simulink model "INDI_POS_SMC_Att"  (R2024b)
settings: Solver=FixedStepDiscrete  StartTime=0.0  StopTime=70  FixedStep=1/250  RelTol=1e-3
values from neighbouring files (symbols this model uses):
  acc_gain = diag([0.5   0.5   0.3  ])    [Parameter.m]
  g = 9.8067    [Parameter.m]
  Jx = 0.005    [Parameter.m]
  Jy = 0.005    [Parameter.m]
  Jz = 0.009    [Parameter.m]
  K2 = 0    [Parameter.m]
  k5 = 0.0388    [Parameter.m]
  k6 = 0.0219    [Parameter.m]
  k7 = 0.3147    [Parameter.m]
  k8 = 0.1244    [Parameter.m]
  l = 0.165    [Parameter.m]
  m = 0.8    [Parameter.m]
  pos_gain = diag([4.14  4.14  3.105])    [Parameter.m]
  Qmax = 0.05    [Parameter.m]
  Tmax = 4    [Parameter.m]
  vel_gain = diag([2.34  2.34  1.77 ])    [Parameter.m]
undefined symbols (not defined in the file or in its folder): DiscIntNeverNeededParam
libraries: simulink x4
settings Model: Creator=user  LastModifiedBy=user
settings DebuggingCC: AlgebraicLoopMsg=none

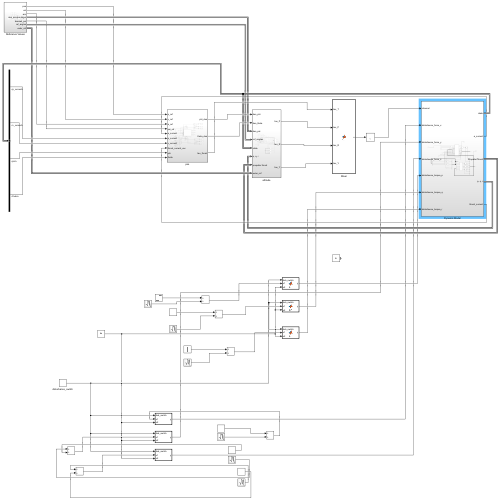
[thumbnail: Simulink's stored preview of the top-level diagram]
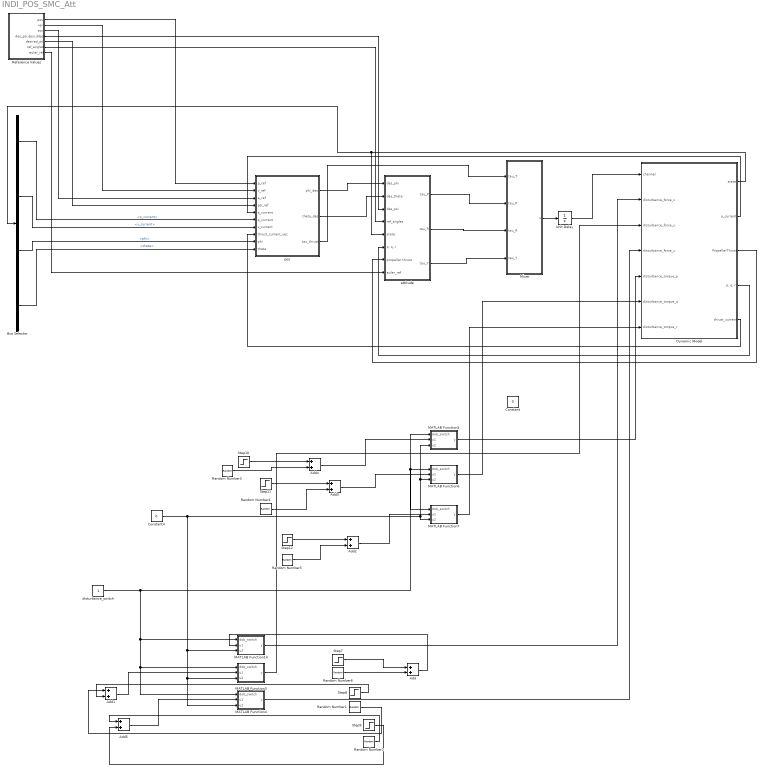
== system INDI_POS_SMC_Att ==
  Add{,1..5} (6 alike) : Sum
  Bus Selector : BusSelector  OutputSignals=p_current,v_current,phi,theta
  Constant : Constant  Value=0
  Constant4 : Constant  Value=0  SampleTime=-1
  Dynamic Model : Subsystem
  MATLAB Function14 : MATLAB Function  TreatAsAtomicUnit=on
  MATLAB Function3 : MATLAB Function  TreatAsAtomicUnit=on
  MATLAB Function4 : MATLAB Function  TreatAsAtomicUnit=on
  MATLAB Function5 : MATLAB Function  TreatAsAtomicUnit=on
  MATLAB Function6 : MATLAB Function  TreatAsAtomicUnit=on
  MATLAB Function7 : MATLAB Function  TreatAsAtomicUnit=on
  Mixer : MATLAB Function  TreatAsAtomicUnit=on
  Random Number{1..6} (6 alike) : RandomNumber  Variance=0.1
  Reference Values : Subsystem
  Step10 : Step  Time=0  After=15
  Step11 : Step  Time=0  After=-15
  Step12 : Step  Time=0  After=2
  Step7 : Step  Time=0
  Step8 : Step  Time=0  After=-0.5
  Step9 : Step  Time=0  After=5
  Unit Delay : UnitDelay  SampleTime=-1  HasFrameUpgradeWarning=on
  attitude : Subsystem
  disturbance_switch : Constant  SampleTime=-1
  pos : Subsystem
  wires:
  Reference Values/1(pos) -> pos/1(p_ref)
  Reference Values/2(vel) -> pos/2(v_ref)
  Reference Values/3(acc) -> pos/3(a_ref)
  Reference Values/5(desired_psi) -> pos/4(psi_ref)
  Bus Selector/1 -> pos/6(p_current)  "<p_current>"
  Bus Selector/2 -> pos/7(v_current)  "<v_current>"
  Reference Values/6(ref_angles) -> attitude/4(ref_angles)
  pos/1(phi_des) -> attitude/1(des_phi)
  pos/2(theta_des) -> attitude/2(des_theta)
  Reference Values/4(des_psi,dpsi,ddpsi) -> attitude/3(des_psi)
  Mixer/1(u) -> Unit Delay/1
  Random Number5/1 -> Add2/2
  Add3/1 -> MATLAB Function6/2(u1)
  Constant4/1 -> MATLAB Function5/3(u2), MATLAB Function6/3(u2), MATLAB Function7/3(u2), MATLAB Function4/3(u2), MATLAB Function3/3(u2), MATLAB Function14/3(u2)
  Step10/1 -> Add4/1
  Add2/1 -> MATLAB Function7/2(u1)
  Random Number4/1 -> Add3/2
  Step11/1 -> Add3/1
  Random Number3/1 -> Add4/2
  disturbance_switch/1 -> MATLAB Function5/1(dob_switch), MATLAB Function7/1(dob_switch), MATLAB Function6/1(dob_switch), MATLAB Function14/1(dob_switch), MATLAB Function4/1(dob_switch), MATLAB Function3/1(dob_switch)
  Add4/1 -> MATLAB Function5/2(u1)
  Step12/1 -> Add2/1
  Step7/1 -> Add/1
  Step8/1 -> Add1/2
  Random Number6/1 -> Add/2
  Step9/1 -> Add5/2
  Add/1 -> MATLAB Function14/2(u1)
  Add1/1 -> MATLAB Function3/2(u1)
  Add5/1 -> MATLAB Function4/2(u1)
  Random Number2/1 -> Add5/1
  Random Number1/1 -> Add1/1
  pos/3(tau_thrust) -> Mixer/1(tau_T)
  attitude/1(tau_P) -> Mixer/2(tau_P)
  attitude/2(tau_R) -> Mixer/3(tau_R)
  attitude/3(tau_Y) -> Mixer/4(tau_Y)
  Dynamic Model/1(state) -> Bus Selector/1, attitude/5(state)
  Dynamic Model/2(a_current) -> pos/5(a_current)
  Dynamic Model/3(PropellerThrust) -> attitude/7(propeller thrust)
  Dynamic Model/4("p, q, r") -> attitude/6("p, q, r")
  Dynamic Model/5(thrust_current) -> pos/8(thrust_current_vec)
  Bus Selector/3 -> pos/9(phi)  "<phi>"
  Bus Selector/4 -> pos/10(theta)  "<theta>"
  MATLAB Function14/1(y) -> Dynamic Model/2(disturbance_force_x)
  MATLAB Function3/1(y) -> Dynamic Model/3(disturbance_force_y)
  MATLAB Function4/1(y) -> Dynamic Model/4(disturbance_force_z)
  MATLAB Function5/1(y) -> Dynamic Model/5(disturbance_torque_p)
  MATLAB Function6/1(y) -> Dynamic Model/6(disturbance_torque_q)
  MATLAB Function7/1(y) -> Dynamic Model/7(disturbance_torque_r)
  Reference Values/7(euler_ref) -> attitude/8(euler_ref)
  Unit Delay/1 -> Dynamic Model/1(channel)

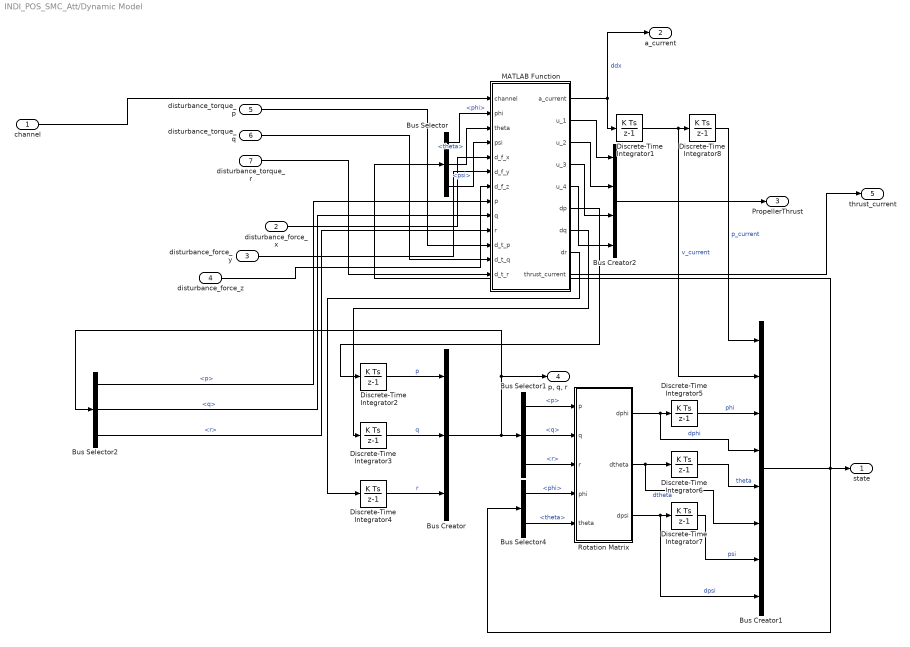
== system INDI_POS_SMC_Att/Dynamic Model ==
  channel : Inport
  disturbance_force_x : Inport  Port=2
  disturbance_force_y : Inport  Port=3
  disturbance_force_z : Inport  Port=4
  disturbance_torque_p : Inport  Port=5
  disturbance_torque_q : Inport  Port=6
  disturbance_torque_r : Inport  Port=7
  Bus Creator : BusCreator  Inputs=3
  Bus Creator1 : BusCreator  Inputs=8
  Bus Creator2 : BusCreator  Inputs=4
  Bus Selector : BusSelector  OutputSignals=phi,theta,psi
  Bus Selector1 : BusSelector  OutputSignals=p,q,r
  Bus Selector2 : BusSelector  OutputSignals=p,q,r
  Bus Selector4 : BusSelector  OutputSignals=phi,theta
  Discrete-Time Integrator{1..8} (8 alike) : DiscreteIntegrator  SampleTime=-1  ICPrevOutput=DiscIntNeverNeededParam  ICPrevScaledInput=DiscIntNeverNeededParam
  MATLAB Function : MATLAB Function  TreatAsAtomicUnit=on
  Rotation Matrix : MATLAB Function  TreatAsAtomicUnit=on
  state : Outport
  a_current : Outport  Port=2
  PropellerThrust : Outport  Port=3
  "p, q, r" : Outport  Port=4
  thrust_current : Outport  Port=5
  wires:
  disturbance_force_y/1 -> MATLAB Function/6(d_f_y)
  disturbance_force_z/1 -> MATLAB Function/7(d_f_z)
  disturbance_force_x/1 -> MATLAB Function/5(d_f_x)
  channel/1 -> MATLAB Function/1(channel)
  Discrete-Time Integrator2/1 -> Bus Creator/1  "p"
  Discrete-Time Integrator3/1 -> Bus Creator/2  "q"
  Discrete-Time Integrator4/1 -> Bus Creator/3  "r"
  Bus Selector2/1 -> MATLAB Function/8(p)  "<p>"
  Bus Selector2/2 -> MATLAB Function/9(q)  "<q>"
  Bus Selector2/3 -> MATLAB Function/10(r)  "<r>"
  Bus Selector1/1 -> Rotation Matrix/1(p)  "<p>"
  Bus Selector1/2 -> Rotation Matrix/2(q)  "<q>"
  Bus Selector1/3 -> Rotation Matrix/3(r)  "<r>"
  Bus Selector4/1 -> Rotation Matrix/4(phi)  "<phi>"
  Bus Selector4/2 -> Rotation Matrix/5(theta)  "<theta>"
  Rotation Matrix/1(dphi) -> Bus Creator1/4, Discrete-Time Integrator5/1  "dphi"
  Rotation Matrix/2(dtheta) -> Bus Creator1/6, Discrete-Time Integrator6/1  "dtheta"
  Rotation Matrix/3(dpsi) -> Bus Creator1/8, Discrete-Time Integrator7/1  "dpsi"
  Discrete-Time Integrator5/1 -> Bus Creator1/3  "phi"
  Discrete-Time Integrator6/1 -> Bus Creator1/5  "theta"
  Discrete-Time Integrator7/1 -> Bus Creator1/7  "psi"
  Discrete-Time Integrator1/1 -> Bus Creator1/2, Discrete-Time Integrator8/1  "v_current"
  Discrete-Time Integrator8/1 -> Bus Creator1/1  "p_current"
  Bus Selector/1 -> MATLAB Function/2(phi)  "<phi>"
  Bus Selector/2 -> MATLAB Function/3(theta)  "<theta>"
  Bus Selector/3 -> MATLAB Function/4(psi)  "<psi>"
  MATLAB Function/2(u_1) -> Bus Creator2/1
  MATLAB Function/3(u_2) -> Bus Creator2/2
  MATLAB Function/4(u_3) -> Bus Creator2/3
  MATLAB Function/5(u_4) -> Bus Creator2/4
  Bus Creator2/1 -> PropellerThrust/1
  disturbance_torque_q/1 -> MATLAB Function/12(d_t_q)
  disturbance_torque_r/1 -> MATLAB Function/13(d_t_r)
  disturbance_torque_p/1 -> MATLAB Function/11(d_t_p)
  MATLAB Function/6(dp) -> Discrete-Time Integrator2/1
  MATLAB Function/7(dq) -> Discrete-Time Integrator3/1
  MATLAB Function/8(dr) -> Discrete-Time Integrator4/1
  Bus Creator/1 -> Bus Selector1/1, Bus Selector2/1, "p, q, r"/1
  Bus Creator1/1 -> Bus Selector/1, Bus Selector4/1, state/1
  MATLAB Function/1(a_current) -> a_current/1, Discrete-Time Integrator1/1  "ddx"
  MATLAB Function/9(thrust_current) -> thrust_current/1

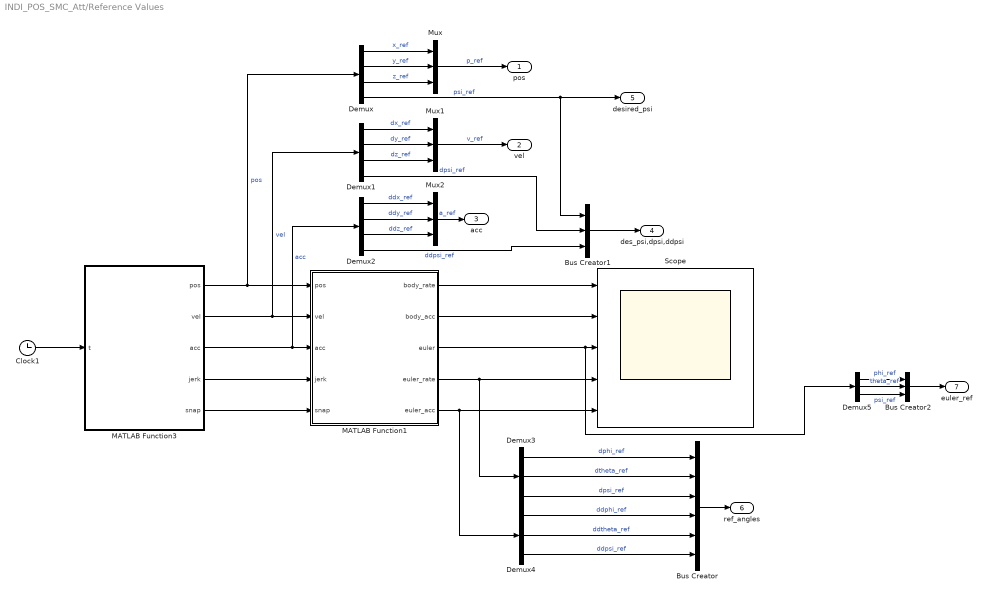
== system INDI_POS_SMC_Att/Reference Values ==
  Bus Creator : BusCreator  Inputs=6
  Bus Creator1 : BusCreator  Inputs=3
  Bus Creator2 : BusCreator  Inputs=3
  Clock1 : Clock
  Demux : Demux
  Demux1 : Demux
  Demux2 : Demux
  Demux3 : Demux  Outputs=3
  Demux4 : Demux  Outputs=3
  Demux5 : Demux  Outputs=3
  MATLAB Function1 : MATLAB Function  TreatAsAtomicUnit=on
  MATLAB Function3 : MATLAB Function  TreatAsAtomicUnit=on
  Mux : Mux  Inputs=3
  Mux1 : Mux  Inputs=3
  Mux2 : Mux  Inputs=3
  Scope : Scope  NumInputPorts=5
  pos : Outport
  vel : Outport  Port=2
  acc : Outport  Port=3
  des_psi,dpsi,ddpsi : Outport  Port=4
  desired_psi : Outport  Port=5
  ref_angles : Outport  Port=6
  euler_ref : Outport  Port=7
  wires:
  MATLAB Function1/3(euler) -> Demux5/1, Scope/3
  MATLAB Function1/5(euler_acc) -> Scope/5, Demux4/1
  Clock1/1 -> MATLAB Function3/1(t)
  MATLAB Function1/1(body_rate) -> Scope/1
  MATLAB Function3/4(jerk) -> MATLAB Function1/4(jerk)
  MATLAB Function1/4(euler_rate) -> Scope/4, Demux3/1
  MATLAB Function3/2(vel) -> Demux1/1, MATLAB Function1/2(vel)  "vel"
  MATLAB Function3/5(snap) -> MATLAB Function1/5(snap)
  MATLAB Function3/3(acc) -> MATLAB Function1/3(acc), Demux2/1  "acc"
  MATLAB Function3/1(pos) -> Demux/1, MATLAB Function1/1(pos)  "pos"
  MATLAB Function1/2(body_acc) -> Scope/2
  Demux3/1 -> Bus Creator/1  "dphi_ref"
  Demux3/2 -> Bus Creator/2  "dtheta_ref"
  Demux/1 -> Mux/1  "x_ref"
  Demux/2 -> Mux/2  "y_ref"
  Demux/3 -> Mux/3  "z_ref"
  Demux/4 -> Bus Creator1/1, desired_psi/1  "psi_ref"
  Demux1/1 -> Mux1/1  "dx_ref"
  Demux1/2 -> Mux1/2  "dy_ref"
  Demux1/3 -> Mux1/3  "dz_ref"
  Demux1/4 -> Bus Creator1/2  "dpsi_ref"
  Demux2/1 -> Mux2/1  "ddx_ref"
  Demux2/2 -> Mux2/2  "ddy_ref"
  Demux2/3 -> Mux2/3  "ddz_ref"
  Demux2/4 -> Bus Creator1/3  "ddpsi_ref"
  Mux/1 -> pos/1  "p_ref"
  Mux1/1 -> vel/1  "v_ref"
  Mux2/1 -> acc/1  "a_ref"
  Demux3/3 -> Bus Creator/3  "dpsi_ref"
  Demux4/1 -> Bus Creator/4  "ddphi_ref"
  Demux4/3 -> Bus Creator/6  "ddpsi_ref"
  Demux4/2 -> Bus Creator/5  "ddtheta_ref"
  Bus Creator/1 -> ref_angles/1
  Bus Creator1/1 -> des_psi,dpsi,ddpsi/1
  Demux5/3 -> Bus Creator2/3  "psi_ref"
  Demux5/1 -> Bus Creator2/1  "phi_ref"
  Demux5/2 -> Bus Creator2/2  "theta_ref"
  Bus Creator2/1 -> euler_ref/1

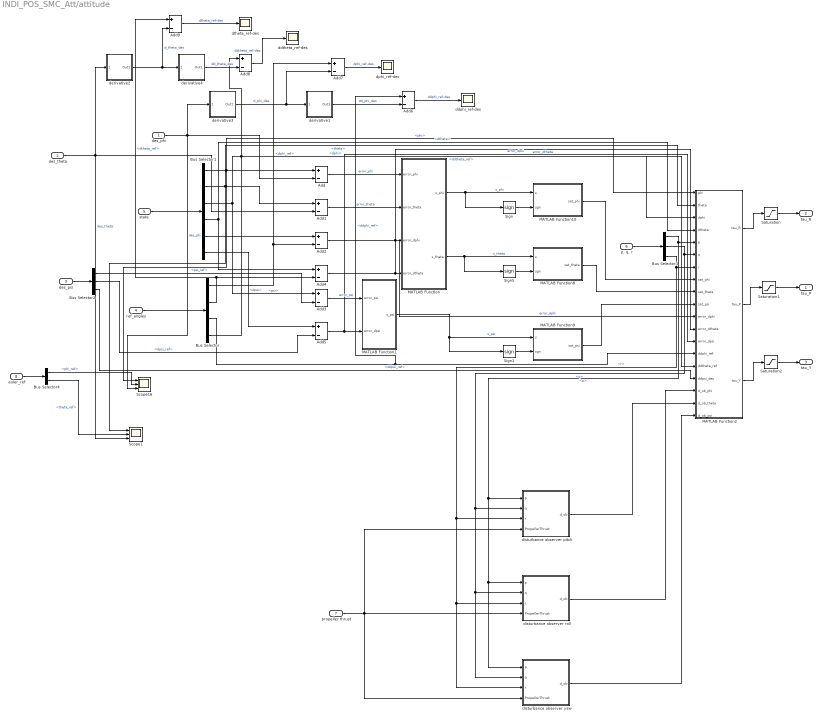
== system INDI_POS_SMC_Att/attitude ==
  des_phi : Inport
  des_theta : Inport  Port=2
  des_psi : Inport  Port=3
  ref_angles : Inport  Port=4
  state : Inport  Port=5
  "p, q, r" : Inport  Port=6
  propeller thrust : Inport  Port=7
  euler_ref : Inport  Port=8
  Add{,1..9} (10 alike) : Sum  Inputs=+-
  Bus Selector : BusSelector  OutputSignals=dphi_ref,dtheta_ref,ddphi_ref,ddtheta_ref
  Bus Selector1 : BusSelector  OutputSignals=phi,theta,dphi,dtheta,psi,dpsi
  Bus Selector2 : BusSelector  OutputSignals=psi_ref,dpsi_ref,ddpsi_ref
  Bus Selector3 : BusSelector  OutputSignals=p,q,r
  Bus Selector4 : BusSelector  OutputSignals=phi_ref,theta_ref
  MATLAB Function : MATLAB Function  TreatAsAtomicUnit=on
  MATLAB Function1 : MATLAB Function  TreatAsAtomicUnit=on
  MATLAB Function10 : MATLAB Function  TreatAsAtomicUnit=on
  MATLAB Function2 : MATLAB Function  TreatAsAtomicUnit=on
  MATLAB Function8 : MATLAB Function  TreatAsAtomicUnit=on
  MATLAB Function9 : MATLAB Function  TreatAsAtomicUnit=on
  Saturation : Saturate  UpperLimit=0.05  LowerLimit=-0.05
  Saturation1 : Saturate  UpperLimit=0.05  LowerLimit=-0.05
  Saturation2 : Saturate  UpperLimit=0.2  LowerLimit=-0.2
  Scope1 : Scope  NumInputPorts=3
  Scope16 : Scope  NumInputPorts=3
  Sign : Signum
  Sign1 : Signum
  Sign5 : Signum
  ddphi_ref-des : Scope
  ddtheta_ref-des : Scope
  derivative1 : Subsystem
  derivative2 : Subsystem
  derivative3 : Subsystem
  derivative4 : Subsystem
  disturbance observer pitch : Subsystem
  disturbance observer roll : Subsystem
  disturbance observer yaw : Subsystem
  dphi_ref-des : Scope
  dtheta_ref-des : Scope
  tau_P : Outport
  tau_R : Outport  Port=2
  tau_Y : Outport  Port=3
  wires:
  ref_angles/1 -> Bus Selector/1
  state/1 -> Bus Selector1/1
  Bus Selector1/1 -> Scope16/1, MATLAB Function2/1(phi), Add/1  "<phi>"
  des_phi/1 -> derivative3/1(des_roll), Scope16/3, Add/2  "des_phi"
  Add/1 -> MATLAB Function/1(error_phi)  "error_phi"
  Bus Selector1/2 -> Scope1/1, MATLAB Function2/2(theta), Add1/1  "<theta>"
  des_theta/1 -> Add1/2, Scope1/3, derivative2/1(des_roll)  "des_theta"
  Add1/1 -> MATLAB Function/2(error_theta)  "error_theta"
  Bus Selector1/3 -> MATLAB Function2/3(dphi), Add2/1  "<dphi>"
  Bus Selector/1 -> Add2/2, Add7/1  "<dphi_ref>"
  Add2/1 -> MATLAB Function/3(error_dphi), MATLAB Function2/11(error_dphi)  "error_dphi"
  Add3/1 -> MATLAB Function1/1(error_psi)  "error_psi"
  Add4/1 -> MATLAB Function2/12(error_dtheta), MATLAB Function/4(error_dtheta)  "error_dtheta"
  Bus Selector1/6 -> Add5/1  "<dpsi>"
  des_psi/1 -> Bus Selector2/1
  Bus Selector2/2 -> Add5/2  "<dpsi_ref>"
  Add5/1 -> MATLAB Function1/2(error_dpsi), MATLAB Function2/13(error_dpsi)  "error_dpsi"
  Bus Selector/3 -> Add6/1, MATLAB Function2/14(ddphi_ref)  "<ddphi_ref>"
  Bus Selector/4 -> Add8/1, MATLAB Function2/15(ddtheta_ref)  "<ddtheta_ref>"
  Bus Selector2/3 -> MATLAB Function2/16(ddpsi_des)  "<ddpsi_ref>"
  Bus Selector1/4 -> MATLAB Function2/4(dtheta), Add4/1  "<dtheta>"
  Bus Selector1/5 -> Add3/1  "<psi>"
  Bus Selector/2 -> Add9/1, Add4/2  "<dtheta_ref>"
  Bus Selector2/1 -> Add3/2  "<psi_ref>"
  MATLAB Function/1(s_phi) -> MATLAB Function10/1(s), Sign/1  "s_phi"
  Sign/1 -> MATLAB Function10/2(sgn)
  MATLAB Function/2(s_theta) -> MATLAB Function8/1(s), Sign5/1  "s_theta"
  Sign5/1 -> MATLAB Function8/2(sgn)
  MATLAB Function1/1(s_psi) -> MATLAB Function9/1(s), Sign1/1  "s_psi"
  Sign1/1 -> MATLAB Function9/2(sgn)
  "p, q, r"/1 -> Bus Selector3/1
  Bus Selector3/1 -> disturbance observer pitch/1("p "), disturbance observer yaw/1("p "), disturbance observer roll/1("p "), MATLAB Function2/5(p)  "<p>"
  Bus Selector3/2 -> disturbance observer pitch/2(q), disturbance observer yaw/2(q), disturbance observer roll/2(q), MATLAB Function2/6(q)  "<q>"
  Bus Selector3/3 -> disturbance observer pitch/3(r), disturbance observer yaw/3(r), disturbance observer roll/3(r), MATLAB Function2/7(r)  "<r>"
  MATLAB Function10/1(sat_phi) -> MATLAB Function2/8(sat_phi)
  MATLAB Function8/1(sat_theta) -> MATLAB Function2/9(sat_theta)
  MATLAB Function9/1(sat_psi) -> MATLAB Function2/10(sat_psi)
  MATLAB Function2/1(tau_R) -> Saturation/1
  MATLAB Function2/2(tau_P) -> Saturation1/1
  MATLAB Function2/3(tau_Y) -> Saturation2/1
  Saturation/1 -> tau_R/1
  Saturation1/1 -> tau_P/1
  Saturation2/1 -> tau_Y/1
  propeller thrust/1 -> disturbance observer pitch/4(PropellerThrust), disturbance observer yaw/4(PropellerThrust), disturbance observer roll/4(PropellerThrust)
  disturbance observer pitch/1(d_ob) -> MATLAB Function2/18(d_ob_theta)
  disturbance observer roll/1(d_ob) -> MATLAB Function2/17(d_ob_phi)
  disturbance observer yaw/1(d_ob) -> MATLAB Function2/19(d_ob_psi)
  derivative3/1(Out1) -> derivative1/1(des_roll), Add7/2  "d_phi_des"
  derivative1/1(Out1) -> Add6/2  "dd_phi_des"
  Add7/1 -> dphi_ref-des/1  "dphi_ref-des"
  Add6/1 -> ddphi_ref-des/1  "ddphi_ref-des"
  derivative2/1(Out1) -> Add9/2, derivative4/1(des_roll)  "d_theta_des"
  derivative4/1(Out1) -> Add8/2  "dd_theta_des"
  Add9/1 -> dtheta_ref-des/1  "dtheta_ref-des"
  Add8/1 -> ddtheta_ref-des/1  "ddtheta_ref-des"
  euler_ref/1 -> Bus Selector4/1
  Bus Selector4/1 -> Scope16/2  "<phi_ref>"
  Bus Selector4/2 -> Scope1/2  "<theta_ref>"

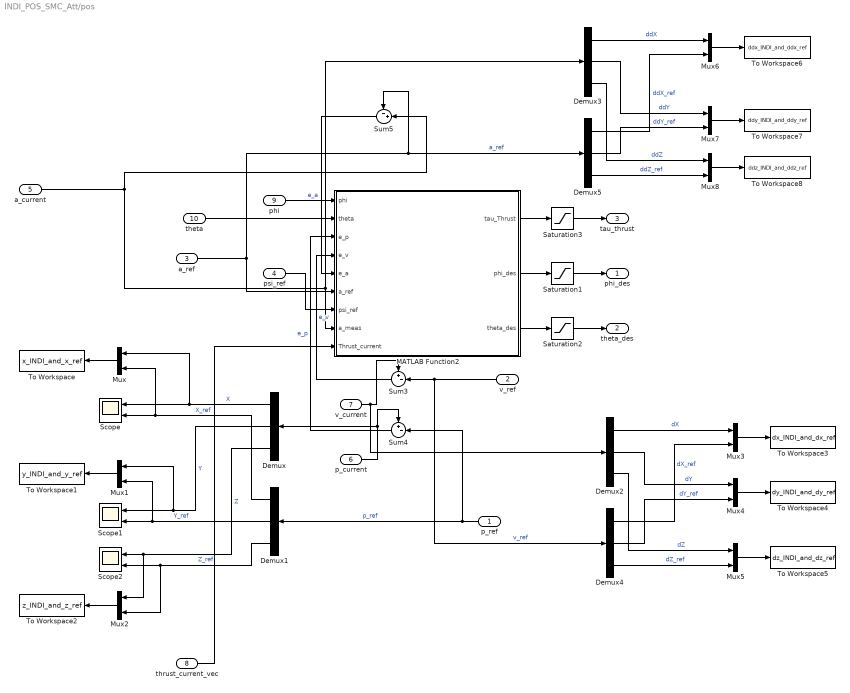
== system INDI_POS_SMC_Att/pos ==
  p_ref : Inport
  v_ref : Inport  Port=2
  a_ref : Inport  Port=3
  psi_ref : Inport  Port=4
  a_current : Inport  Port=5
  p_current : Inport  Port=6
  v_current : Inport  Port=7
  thrust_current_vec : Inport  Port=8
  phi : Inport  Port=9
  theta : Inport  Port=10
  Demux{,1..5} (6 alike) : Demux  Outputs=3
  MATLAB Function2 : MATLAB Function  TreatAsAtomicUnit=on
  Mux{,1..8} (9 alike) : Mux  Inputs=2
  Saturation1 : Saturate  UpperLimit=0.8727  LowerLimit=-0.8727
  Saturation2 : Saturate  UpperLimit=0.8727  LowerLimit=-0.8727
  Saturation3 : Saturate  UpperLimit=1.7  LowerLimit=1
  Scope : Scope  NumInputPorts=2
  Scope1 : Scope  NumInputPorts=2
  Scope2 : Scope  NumInputPorts=2
  Sum3 : Sum  Inputs=+-|
  Sum4 : Sum  Inputs=+-|
  Sum5 : Sum  Inputs=-+|
  To Workspace : ToWorkspace  VariableName=x_INDI_and_x_ref  SaveFormat=Timeseries  SampleTime=-1
  To Workspace1 : ToWorkspace  VariableName=y_INDI_and_y_ref  SaveFormat=Timeseries  SampleTime=-1
  To Workspace2 : ToWorkspace  VariableName=z_INDI_and_z_ref  SaveFormat=Timeseries  SampleTime=-1
  To Workspace3 : ToWorkspace  VariableName=dx_INDI_and_dx_ref  SaveFormat=Timeseries  SampleTime=-1
  To Workspace4 : ToWorkspace  VariableName=dy_INDI_and_dy_ref  SaveFormat=Timeseries  SampleTime=-1
  To Workspace5 : ToWorkspace  VariableName=dz_INDI_and_dz_ref  SaveFormat=Timeseries  SampleTime=-1
  To Workspace6 : ToWorkspace  VariableName=ddx_INDI_and_ddx_ref  SaveFormat=Timeseries  SampleTime=-1
  To Workspace7 : ToWorkspace  VariableName=ddy_INDI_and_ddy_ref  SaveFormat=Timeseries  SampleTime=-1
  To Workspace8 : ToWorkspace  VariableName=ddz_INDI_and_ddz_ref  SaveFormat=Timeseries  SampleTime=-1
  phi_des : Outport
  theta_des : Outport  Port=2
  tau_thrust : Outport  Port=3
  wires:
  p_ref/1 -> Demux1/1, Sum4/2  "p_ref"
  a_ref/1 -> Demux5/1, Sum5/1, MATLAB Function2/6(a_ref)  "a_ref"
  Demux/1 -> Scope/1, Mux/1  "X"
  Demux/2 -> Mux1/1, Scope1/1  "Y"
  Demux/3 -> Mux2/1, Scope2/1  "Z"
  Demux1/3 -> Scope2/2, Mux2/2  "Z_ref"
  Demux1/2 -> Mux1/2, Scope1/2  "Y_ref"
  Demux1/1 -> Mux/2, Scope/2  "X_ref"
  v_ref/1 -> Demux4/1, Sum3/2  "v_ref"
  Sum3/1 -> MATLAB Function2/4(e_v)  "e_v"
  Sum4/1 -> MATLAB Function2/3(e_p)  "e_p"
  Sum5/1 -> MATLAB Function2/5(e_a)  "e_a"
  psi_ref/1 -> MATLAB Function2/7(psi_ref)
  MATLAB Function2/2(phi_des) -> Saturation1/1
  MATLAB Function2/3(theta_des) -> Saturation2/1
  Demux2/1 -> Mux3/1  "dX"
  Demux2/2 -> Mux4/1  "dY"
  Demux2/3 -> Mux5/1  "dZ"
  Demux3/1 -> Mux6/1  "ddX"
  Demux3/2 -> Mux7/1  "ddY"
  Demux3/3 -> Mux8/1  "ddZ"
  Mux/1 -> To Workspace/1
  Mux1/1 -> To Workspace1/1
  Mux2/1 -> To Workspace2/1
  Demux4/1 -> Mux3/2  "dX_ref"
  Demux4/2 -> Mux4/2  "dY_ref"
  Demux4/3 -> Mux5/2  "dZ_ref"
  Mux3/1 -> To Workspace3/1
  Mux4/1 -> To Workspace4/1
  Mux5/1 -> To Workspace5/1
  Mux6/1 -> To Workspace6/1
  Demux5/1 -> Mux6/2  "ddX_ref"
  Demux5/2 -> Mux7/2  "ddY_ref"
  Demux5/3 -> Mux8/2  "ddZ_ref"
  Mux7/1 -> To Workspace7/1
  Mux8/1 -> To Workspace8/1
  MATLAB Function2/1(tau_Thrust) -> Saturation3/1
  a_current/1 -> Sum5/2, Demux3/1, MATLAB Function2/8(a_meas)
  v_current/1 -> Demux2/1, Sum3/1
  p_current/1 -> Demux/1, Sum4/1
  thrust_current_vec/1 -> MATLAB Function2/9(Thrust_current)
  Saturation1/1 -> phi_des/1
  Saturation2/1 -> theta_des/1
  Saturation3/1 -> tau_thrust/1
  phi/1 -> MATLAB Function2/1(phi)
  theta/1 -> MATLAB Function2/2(theta)

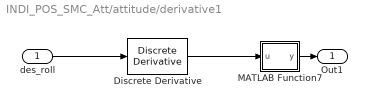
== system INDI_POS_SMC_Att/attitude/derivative1 ==
  des_roll : Inport
  Discrete Derivative : simulink/Discrete/Discrete Derivative  gainval=1.0  ICPrevScaledInput=0.0  OutMin=[]  OutMax=[]  OutDataType=fixdt(1, 16)  OutScaling=2^-10  DoSatur=off
  MATLAB Function7 : MATLAB Function  TreatAsAtomicUnit=on
  Out1 : Outport
  wires:
  des_roll/1 -> Discrete Derivative/1
  MATLAB Function7/1(y) -> Out1/1
  Discrete Derivative/1 -> MATLAB Function7/1(u)

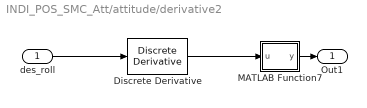
== system INDI_POS_SMC_Att/attitude/derivative2 ==
  des_roll : Inport
  Discrete Derivative : simulink/Discrete/Discrete Derivative  gainval=1.0  ICPrevScaledInput=0.0  OutMin=[]  OutMax=[]  OutDataType=fixdt(1, 16)  OutScaling=2^-10  DoSatur=off
  MATLAB Function7 : MATLAB Function  TreatAsAtomicUnit=on
  Out1 : Outport
  wires:
  des_roll/1 -> Discrete Derivative/1
  MATLAB Function7/1(y) -> Out1/1
  Discrete Derivative/1 -> MATLAB Function7/1(u)

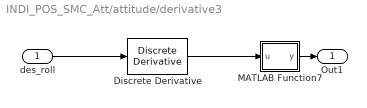
== system INDI_POS_SMC_Att/attitude/derivative3 ==
  des_roll : Inport
  Discrete Derivative : simulink/Discrete/Discrete Derivative  gainval=1.0  ICPrevScaledInput=0.0  OutMin=[]  OutMax=[]  OutDataType=fixdt(1, 16)  OutScaling=2^-10  DoSatur=off
  MATLAB Function7 : MATLAB Function  TreatAsAtomicUnit=on
  Out1 : Outport
  wires:
  des_roll/1 -> Discrete Derivative/1
  MATLAB Function7/1(y) -> Out1/1
  Discrete Derivative/1 -> MATLAB Function7/1(u)

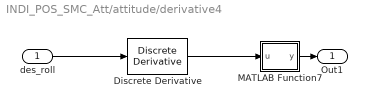
== system INDI_POS_SMC_Att/attitude/derivative4 ==
  des_roll : Inport
  Discrete Derivative : simulink/Discrete/Discrete Derivative  gainval=1.0  ICPrevScaledInput=0.0  OutMin=[]  OutMax=[]  OutDataType=fixdt(1, 16)  OutScaling=2^-10  DoSatur=off
  MATLAB Function7 : MATLAB Function  TreatAsAtomicUnit=on
  Out1 : Outport
  wires:
  des_roll/1 -> Discrete Derivative/1
  MATLAB Function7/1(y) -> Out1/1
  Discrete Derivative/1 -> MATLAB Function7/1(u)

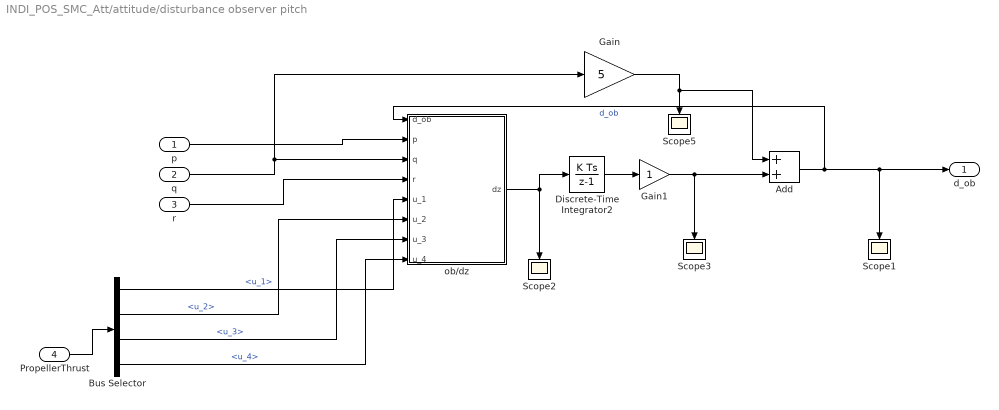
== system INDI_POS_SMC_Att/attitude/disturbance observer pitch ==
  "p " : Inport
  q : Inport  Port=2
  r : Inport  Port=3
  PropellerThrust : Inport  Port=4
  Add : Sum
  Bus Selector : BusSelector  OutputSignals=u_1,u_2,u_3,u_4
  Discrete-Time Integrator2 : DiscreteIntegrator  SampleTime=-1  ICPrevOutput=DiscIntNeverNeededParam  ICPrevScaledInput=DiscIntNeverNeededParam
  Gain : Gain  Gain=5
  Gain1 : Gain
  Scope{1..3,5} (4 alike) : Scope
  ob/dz : MATLAB Function  TreatAsAtomicUnit=on
  d_ob : Outport
  wires:
  ob/dz/1(dz) -> Discrete-Time Integrator2/1, Scope2/1
  Discrete-Time Integrator2/1 -> Gain1/1
  Gain/1 -> Scope5/1, Add/1
  Add/1 -> Scope1/1, d_ob/1, ob/dz/1(d_ob)  "d_ob"
  Gain1/1 -> Add/2, Scope3/1
  r/1 -> ob/dz/4(r)
  q/1 -> ob/dz/3(q), Gain/1
  "p "/1 -> ob/dz/2(p)
  PropellerThrust/1 -> Bus Selector/1
  Bus Selector/1 -> ob/dz/5(u_1)  "<u_1>"
  Bus Selector/2 -> ob/dz/6(u_2)  "<u_2>"
  Bus Selector/3 -> ob/dz/7(u_3)  "<u_3>"
  Bus Selector/4 -> ob/dz/8(u_4)  "<u_4>"

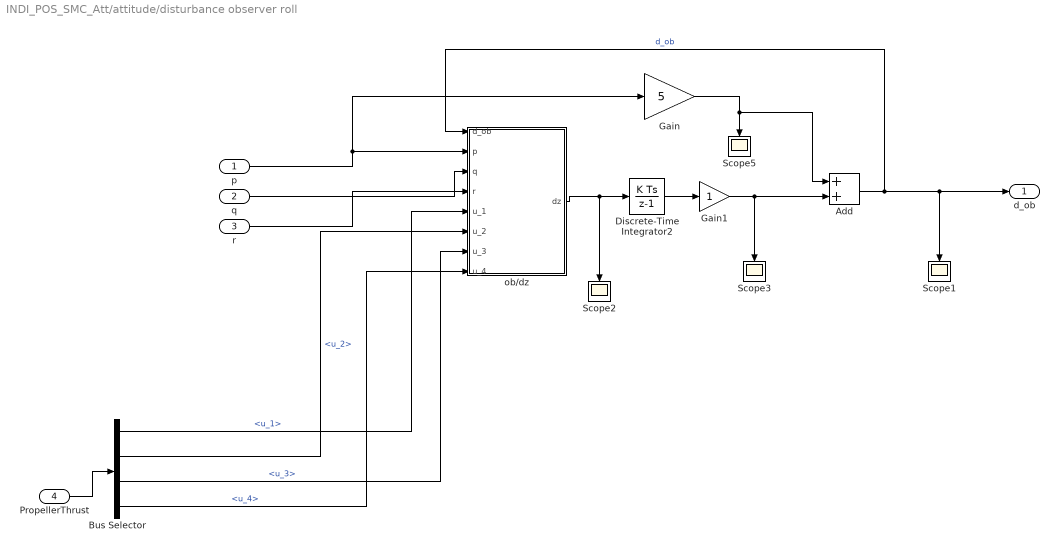
== system INDI_POS_SMC_Att/attitude/disturbance observer roll ==
  "p " : Inport
  q : Inport  Port=2
  r : Inport  Port=3
  PropellerThrust : Inport  Port=4
  Add : Sum
  Bus Selector : BusSelector  OutputSignals=u_1,u_2,u_3,u_4
  Discrete-Time Integrator2 : DiscreteIntegrator  SampleTime=-1  ICPrevOutput=DiscIntNeverNeededParam  ICPrevScaledInput=DiscIntNeverNeededParam
  Gain : Gain  Gain=5
  Gain1 : Gain
  Scope{1..3,5} (4 alike) : Scope
  ob/dz : MATLAB Function  TreatAsAtomicUnit=on
  d_ob : Outport
  wires:
  ob/dz/1(dz) -> Discrete-Time Integrator2/1, Scope2/1
  Discrete-Time Integrator2/1 -> Gain1/1
  Gain/1 -> Scope5/1, Add/1
  Add/1 -> Scope1/1, d_ob/1, ob/dz/1(d_ob)  "d_ob"
  Gain1/1 -> Add/2, Scope3/1
  r/1 -> ob/dz/4(r)
  q/1 -> ob/dz/3(q)
  "p "/1 -> Gain/1, ob/dz/2(p)
  Bus Selector/4 -> ob/dz/8(u_4)  "<u_4>"
  Bus Selector/3 -> ob/dz/7(u_3)  "<u_3>"
  Bus Selector/1 -> ob/dz/5(u_1)  "<u_1>"
  PropellerThrust/1 -> Bus Selector/1
  Bus Selector/2 -> ob/dz/6(u_2)  "<u_2>"

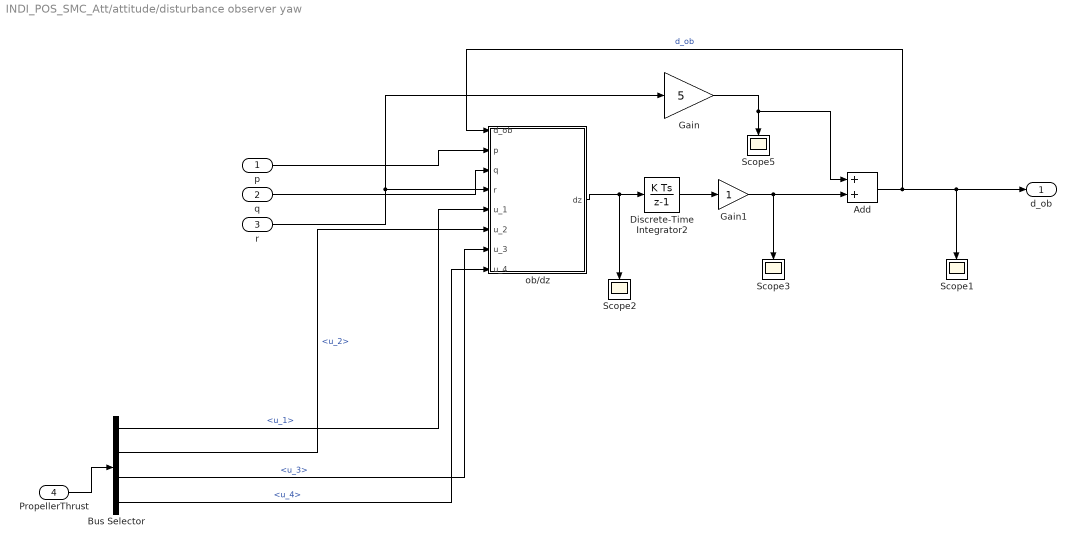
== system INDI_POS_SMC_Att/attitude/disturbance observer yaw ==
  "p " : Inport
  q : Inport  Port=2
  r : Inport  Port=3
  PropellerThrust : Inport  Port=4
  Add : Sum
  Bus Selector : BusSelector  OutputSignals=u_1,u_2,u_3,u_4
  Discrete-Time Integrator2 : DiscreteIntegrator  SampleTime=-1  ICPrevOutput=DiscIntNeverNeededParam  ICPrevScaledInput=DiscIntNeverNeededParam
  Gain : Gain  Gain=5
  Gain1 : Gain
  Scope{1..3,5} (4 alike) : Scope
  ob/dz : MATLAB Function  TreatAsAtomicUnit=on
  d_ob : Outport
  wires:
  ob/dz/1(dz) -> Discrete-Time Integrator2/1, Scope2/1
  Discrete-Time Integrator2/1 -> Gain1/1
  Gain/1 -> Scope5/1, Add/1
  Add/1 -> Scope1/1, d_ob/1, ob/dz/1(d_ob)  "d_ob"
  Gain1/1 -> Add/2, Scope3/1
  r/1 -> Gain/1, ob/dz/4(r)
  q/1 -> ob/dz/3(q)
  "p "/1 -> ob/dz/2(p)
  Bus Selector/4 -> ob/dz/8(u_4)  "<u_4>"
  Bus Selector/3 -> ob/dz/7(u_3)  "<u_3>"
  Bus Selector/1 -> ob/dz/5(u_1)  "<u_1>"
  PropellerThrust/1 -> Bus Selector/1
  Bus Selector/2 -> ob/dz/6(u_2)  "<u_2>"

== matlab function INDI_POS_SMC_Att/attitude/derivative1/MATLAB Function7 ==
  data: u input; y output
function y = fcn(u)
if abs(u)>30 
    u=0;
end
y = u;

== matlab function INDI_POS_SMC_Att/attitude/derivative2/MATLAB Function7 ==
  data: u input; y output
function y = fcn(u)
if abs(u)>30 
    u=0;
end
y = u;

== matlab function INDI_POS_SMC_Att/attitude/MATLAB Function ==
  data: error_phi input; s_phi output; s_theta output; error_theta input; error_dphi input; error_dtheta input; a3 parameter
function [s_phi, s_theta] = sliding_surface(error_phi, error_theta, error_dphi, error_dtheta, a3)


s_phi = ((a3 * error_phi) + error_dphi) / 0.5;
s_theta = ((a3 * error_theta) + error_dtheta) / 0.5;
end

== matlab function INDI_POS_SMC_Att/attitude/derivative4/MATLAB Function7 ==
  data: u input; y output
function y = fcn(u)
if abs(u)>30 
    u=0;
end
y = u;

== matlab function INDI_POS_SMC_Att/attitude/derivative3/MATLAB Function7 ==
  data: u input; y output
function y = fcn(u)
if abs(u)>30 
    u=0;
end
y = u;

== matlab function INDI_POS_SMC_Att/attitude/MATLAB Function1 ==
  data: error_psi input; s_psi output; error_dpsi input; a4 parameter
function s_psi = fcn(error_psi, error_dpsi, a4)

s_psi = ((a4 * error_psi) + error_dpsi) / 0.5;

end

== matlab function INDI_POS_SMC_Att/Dynamic Model/MATLAB Function ==
  data: channel input; a_current output size=[3 1]; phi input; theta input; psi input; d_f_x input; d_f_y input; d_f_z input; u_1 output size=1; u_2 output size=1; u_3 output size=1; u_4 output size=1; p input; q input; r input; d_t_p input; d_t_q input; d_t_r input; dp output size=1; dq output size=1; dr output size=1; thrust_current output size=[3 1]; m parameter; l parameter; g parameter; K2 parameter; Tmax parameter; Jx parameter; Jy parameter; Jz parameter; Qmax parameter
function [a_current, u_1, u_2, u_3, u_4, dp, dq, dr, thrust_current] = fcn(channel, phi, theta, psi, d_f_x, d_f_y, d_f_z, p, q, r, d_t_p, d_t_q, d_t_r, m, l, g, K2, Tmax, Jx, Jy, Jz, Qmax)

z_W = [0; 0; 1];

% PWM_max = 2000;
% PWM_min = 1000;

% for index = 1:4
%     if channel(index) < PWM_min
%         channel(index) = PWM_min;
%     elseif channel(index) > PWM_max
%         channel(index) = PWM_max;
%     end
% end
% 
% u_1 = (channel(1) - PWM_min) / (PWM_max - PWM_min);
% u_2 = (channel(2) - PWM_min) / (PWM_max - PWM_min);
% u_3 = (channel(3) - PWM_min) / (PWM_max - PWM_min);
% u_4 = (channel(4) - PWM_min) / (PWM_max - PWM_min);

u_1 = channel(1);
u_2 = channel(2);
u_3 = channel(3);
u_4 = channel(4);

thrust_total = Tmax * (u_1 + u_2 + u_3 + u_4);

s_phi = sin (phi);
c_phi = cos (phi);
s_th = sin (theta);
c_th = cos (theta);
s_psi = sin (psi);
c_psi = cos (psi);

one = (c_psi * s_th * c_phi) + (s_psi * s_phi);
two = (s_psi * s_th * c_phi) - (c_psi * s_phi);
three = c_th * c_phi;

z_B = [one; two; three];

f_ext = [d_f_x; d_f_y; d_f_z];
a_current = ((thrust_total * z_B) - (m * g * z_W) + f_ext) / m;
thrust_current = thrust_total * z_B;

dp = (-Tmax*(u_1*(l*sqrt(2)/2)+ u_4*(l*sqrt(2)/2)- u_2*(l*sqrt(2)/2)- u_3*(l*sqrt(2)/2)) - K2*p*abs(p) - q*r*(Jz-Jy))/Jx + d_t_p;
dq = (-Tmax*(u_2*(l*sqrt(2)/2)+ u_4*(l*sqrt(2)/2)- u_1*(l*sqrt(2)/2)- u_3*(l*sqrt(2)/2)) - K2*q*abs(q) - p*r*(Jx-Jz))/Jy + d_t_q;
dr = (Qmax*(u_1+u_2-u_3-u_4) - K2*r*abs(r) - p*q*(Jy-Jx))/Jz + d_t_r;
end

== matlab function INDI_POS_SMC_Att/attitude/MATLAB Function2 ==
  data: tau_R output; tau_P output; tau_Y output; phi input; theta input; dphi input; dtheta input; p input; q input; r input; sat_phi input; sat_theta input; sat_psi input; error_dphi input; error_dtheta input; error_dpsi input; ddphi_ref input; ddtheta_ref input; ddpsi_des input; d_ob_phi input; d_ob_theta input; d_ob_psi input; k5 parameter; k6 parameter; k7 parameter; k8 parameter; l parameter; Jx parameter; Jy parameter; Jz parameter; K2 parameter; Tmax parameter; Qmax parameter
function [tau_R, tau_P, tau_Y] = fcn(phi, theta, dphi, dtheta, p, q, r, sat_phi, sat_theta, sat_psi, error_dphi, error_dtheta, error_dpsi, ddphi_ref, ddtheta_ref, ddpsi_des, d_ob_phi, d_ob_theta, d_ob_psi, k5, k6, k7, k8, l, Jx, Jy, Jz, K2, Tmax, Qmax)

f_phi1 = q*((1/cos(theta)^2)*dtheta*sin(phi)+tan(theta)*cos(phi)*dphi)+r*((1/cos(theta)^2)*dtheta*cos(phi)-tan(theta)*sin(phi)*dphi);
f_phi = f_phi1-((Jz-Jy)/Jx)*q*r-K2*p*abs(p)/Jx-((Jx-Jz)/Jy)*p*r*tan(theta)*sin(phi)-K2*q*abs(q)*tan(theta)*sin(phi)/Jy-((Jy-Jx)/Jz)*p*q*tan(theta)*cos(phi)-K2*r*abs(r)*tan(theta)*cos(phi)/Jz;
f_theta1 = -(q*sin(phi)*dphi+r*cos(phi)*dphi);
f_theta = f_theta1-(((Jx-Jz)/Jy)*p*r*cos(phi)+K2*q*abs(q)*cos(phi)/Jy-((Jy-Jx)/Jz)*p*q*sin(phi)-K2*r*abs(r)*sin(phi)/Jz);
f_psi1 = q*(cos(phi)*dphi*cos(theta)+sin(phi)*sin(theta)*dtheta)/cos(theta)^2+r*(cos(phi)*sin(theta)*dtheta-sin(phi)*dphi*cos(theta))/cos(theta)^2;
f_psi = f_psi1-cos(phi)*(Jy-Jx)*q*p/(cos(theta)*Jz)-(cos(phi)*K2*r*abs(r))/(cos(theta)*Jz)-(sin(phi)*(Jx-Jz)*p*r)/(cos(theta)*Jy)-(sin(phi)*K2*q*abs(q))/(cos(theta)*Jy);

A = [ 1, Jx*tan(theta)*sin(phi)/Jy, -(Jx*4*Qmax*tan(theta)*cos(phi))/(Jz*2*l*sqrt(2)*Tmax);
    0, 1, (Jy*tan(phi)*4*Qmax)/(Jz*2*l*sqrt(2)*Tmax);
    0, -(Jz*tan(phi)*2*l*sqrt(2)*Tmax)/(Jy*4*Qmax), 1 ];
B = [k5*sat_phi+k6*error_dphi+Jx*(f_phi-ddphi_ref)/(2*l*sqrt(2)*Tmax);
    k5*sat_theta/cos(phi)+(k6/cos(phi))*error_dtheta+Jy*(f_theta-ddtheta_ref)/(2*l*sqrt(2)*Tmax*cos(phi));
    -k7*sat_psi*(cos(theta)/cos(phi))-k8*(cos(theta)/cos(phi))*error_dpsi-cos(theta)*Jz*(f_psi-ddpsi_des)/(4*Qmax*cos(phi))];

taus = linsolve(A,B);

tau_R = taus(1)+(d_ob_phi)*Jx/(Tmax*2*l*sqrt(2));
tau_P = taus(2)+(d_ob_theta)*Jy/(Tmax*2*l*sqrt(2));
tau_Y = taus(3)-d_ob_psi*Jz/(Qmax*4);

end

== matlab function INDI_POS_SMC_Att/Dynamic Model/Rotation Matrix ==
  data: p input; dphi output; dtheta output; dpsi output; q input; r input; phi input; theta input
function [dphi,dtheta,dpsi] = fcn(p,q,r,phi,theta)

%roll
dphi=p+q*sin(phi)*tan(theta)+r*cos(phi)*tan(theta);

%pitch
dtheta=q*cos(phi)-r*sin(phi);

%yaw
dpsi=q*sin(phi)/cos(theta)+r*cos(phi)/cos(theta);
% dphi=p
% dtheta=q
% dpsi=r

== matlab function INDI_POS_SMC_Att/attitude/disturbance observer pitch/ob//dz ==
  data: d_ob input; p input; dz output; q input; r input; u_1 input; u_2 input; u_3 input; u_4 input
 function dz  = fcn(d_ob, p, q, r, u_1, u_2, u_3, u_4)

% dz = -k_ob*d_ob - k_ob/Jy*(-T_max*l*sqrt(2)/2*(4*tau_Pitch)-K_2*q-p*r*(Jx-Jz));
T_max = 4;
K_4 = 0;
k_ob = 5;

l = 0.165;
Jx = 0.005; 
Jy = 0.005;
Jz = 0.009;

dz = -k_ob*d_ob - k_ob/Jy*(-T_max*(u_2*(l*sqrt(2)/2)+ u_4*(l*sqrt(2)/2)- u_1*(l*sqrt(2)/2)- u_3*(l*sqrt(2)/2))-K_4*q*abs(q)-p*r*(Jx-Jz));

end

== matlab function INDI_POS_SMC_Att/attitude/disturbance observer roll/ob//dz ==
  data: d_ob input; p input; dz output; q input; r input; u_1 input; u_2 input; u_3 input; u_4 input
 function dz  = fcn(d_ob, p, q, r, u_1, u_2, u_3, u_4)

l = 0.165;
Jx = 0.005; 
Jy = 0.005;
Jz = 0.009;

T_max = 4;
K_4 = 0;
k_ob = 5;

dz = -k_ob*d_ob - k_ob/Jx*(-T_max*(u_1*(l*sqrt(2)/2)+ u_4*(l*sqrt(2)/2)- u_2*(l*sqrt(2)/2)- u_3*(l*sqrt(2)/2))-K_4*p*abs(p)-q*r*(Jz-Jy));
end

== matlab function INDI_POS_SMC_Att/attitude/disturbance observer yaw/ob//dz ==
  data: d_ob input; p input; dz output; q input; r input; u_1 input; u_2 input; u_3 input; u_4 input
 function dz  = fcn(d_ob, p, q, r, u_1, u_2, u_3, u_4)

 l = 0.165;
Jx = 0.005; 
Jy = 0.005;
Jz = 0.009;
Q_max = 0.05;
k_ob = 5;
K_4 = 0;
% k_ob=0.1;
% dz = -k_ob*d_ob - k_ob/Jz*(Q_max*(4*tau_Yaw)-K_2*r-q*p*(Jy-Jx));
dz = -k_ob*d_ob - k_ob/Jz*(Q_max*(u_1+u_2-u_3-u_4)-K_4*r*abs(r)-q*p*(Jy-Jx));
end

== matlab function INDI_POS_SMC_Att/attitude/MATLAB Function8 ==
  data: s input; sgn input; sat_theta output
function sat_theta = fcn( s, sgn )
% sat_theta=2/(1+exp(-s))-1;
if  abs(s)< 1
sat_theta = s;
else
sat_theta = sgn;
end

== matlab function INDI_POS_SMC_Att/attitude/MATLAB Function9 ==
  data: s input; sgn input; sat_psi output
function sat_psi = fcn( s, sgn )
% sat_psi=2/(1+exp(-s))-1;
if  abs(s)< 1
sat_psi = s;
else
sat_psi = sgn;
end

== matlab function INDI_POS_SMC_Att/attitude/MATLAB Function10 ==
  data: s input; sgn input; sat_phi output
function sat_phi = fcn( s, sgn )
% sat_phi=2/(1+exp(-s))-1;
if  abs(s)< 1
sat_phi = s;
else
sat_phi = sgn;
end

== matlab function INDI_POS_SMC_Att/MATLAB Function14 ==
  data: dob_switch input; y output; u1 input; u2 input
function y = fcn(dob_switch,u1,u2)
y=0;
if dob_switch == 1
    y = u1;
elseif dob_switch ==0
    y=u2;
 
end

== matlab function INDI_POS_SMC_Att/MATLAB Function3 ==
  data: dob_switch input; y output; u1 input; u2 input
function y = fcn(dob_switch,u1,u2)
y=0;
if dob_switch == 1
    y = u1;
elseif dob_switch ==0
    y=u2;
 
end

== matlab function INDI_POS_SMC_Att/MATLAB Function4 ==
  data: dob_switch input; y output; u1 input; u2 input
function y = fcn(dob_switch,u1,u2)
y=0;
if dob_switch == 1
    y = u1;
elseif dob_switch ==0
    y=u2;
 
end

== matlab function INDI_POS_SMC_Att/MATLAB Function5 ==
  data: dob_switch input; y output; u1 input; u2 input
function y = fcn(dob_switch,u1,u2)
y=0;
if dob_switch == 1
    y = u1;
elseif dob_switch ==0
    y=u2;
 
end

== matlab function INDI_POS_SMC_Att/MATLAB Function6 ==
  data: dob_switch input; y output; u1 input; u2 input
function y = fcn(dob_switch,u1,u2)
y=0;
if dob_switch == 1
    y = u1;
elseif dob_switch ==0
    y=u2;
 
end

== matlab function INDI_POS_SMC_Att/MATLAB Function7 ==
  data: dob_switch input; y output; u1 input; u2 input
function y = fcn(dob_switch,u1,u2)
y=0;
if dob_switch == 1
    y = u1;
elseif dob_switch ==0
    y=u2;
 
end

== matlab function INDI_POS_SMC_Att/Reference Values/MATLAB Function1 ==
  data: pos input; body_rate output; vel input; acc input; jerk input; snap input; body_acc output; euler output; euler_rate output; euler_acc output
function [body_rate, body_acc, euler, euler_rate, euler_acc] = diff_flat (pos, vel, acc, jerk, snap)

    g = 9.80665;
    m = 0.8;
    
    x = pos (1);
    y = pos (2);
    z = pos (3);
    psi = pos (4);

    dx = vel (1);
    dy = vel (2);
    dz = vel (3);
    d_psi = vel (4);

    ddx = acc (1);
    ddy = acc (2);
    ddz = acc (3);
    dd_psi = acc (4);
       
    j_x = jerk (1);
    j_y = jerk (2);
    j_z = jerk (3);
    psi3 = jerk (4);

    snap_x = snap (1);
    snap_y = snap (2);
    snap_z = snap (3);
    psi4 = snap (4);


    s_x = sin (x);
    c_x = cos (x);
    s_y = sin (y);
    c_y = cos (y);
    s_psi = sin (psi);
    c_psi = cos (psi);

    ddx2 = ddx ^2;
    ddy2 = ddy ^2;
    ddz2 = (ddz + g) ^2;

    term = (s_psi * ddx) - (c_psi * ddy);
    term2 = term ^2;
    
    secterm = (s_psi * ddy) + (c_psi * ddx);

    nu = sqrt ((ddx2 + ddy2 + ddz2) * (ddz2 + term2));

    eta = sqrt (ddz2 + term2);

    kappa = sqrt (ddx2 + ddy2 + ddz2);

    w_R_b = zeros (3, 3);

    w_R_b (1, 1) = ((c_psi * ddz2) - (term * ddy)) / nu;
    w_R_b (1, 2) = -(s_psi * (ddz + g)) / eta;
    w_R_b (1, 3) = ddx / kappa;

    w_R_b (2, 1) = ((s_psi * ddz2) + (term * ddx)) / nu;
    w_R_b (2, 2) = (c_psi * (ddz + g)) / eta;
    w_R_b (2, 3) = ddy / kappa;
    
    w_R_b (3, 1) = - ((ddz + g) * secterm) / nu;
    w_R_b (3, 2) = term / eta;
    w_R_b (3, 3) = (ddz + g) / kappa;

    theta = atan2 (secterm, eta);
    phi = atan2 (term, ddz + g);

    s_phi = sin (phi);
    c_phi = cos (phi);
    s_theta = sin (theta);
    c_theta = cos (theta);

    u1 = m * sqrt (ddx2 + ddy2 + ddz2);

    p = (-m / u1) * ((w_R_b (1, 2) * j_x) + (w_R_b (2, 2) * j_y) + (w_R_b (3, 2) * j_z));
    q = (m / u1) * ((w_R_b (1, 1) * j_x) + (w_R_b (2, 1) * j_y) + (w_R_b (3, 1) * j_z));
   
    d_phi = (p + (c_phi * s_theta * d_psi)) / c_theta;
    d_theta = q - (s_phi * d_psi);

    r = (s_theta * d_phi) + (c_phi * c_theta * d_psi);    

    front = m / u1;
    one = ((w_R_b (1, 2) * snap_x) + (w_R_b (2, 2) * snap_y) + (w_R_b (3, 2) * snap_z));
    two = 2 * ((ddx * j_x) + (ddy * j_y) + ((ddz + g) * j_z)) / kappa;
    d_p = -(front * (one + (p * two))) + (r * q);
    three = ((w_R_b (1, 1) * snap_x) + (w_R_b (2, 1) * snap_y) + (w_R_b (3, 1) * snap_z));
    d_q = (front * (three - (q * two))) - (r * p);

    a_ready = zeros (3, 3);
    a_ready (1, 1) = c_psi;
    a_ready (2, 1) = s_psi;
    a_ready (1, 2) = -(s_psi * (ddz + g)) / eta;
    a_ready (2, 2) = (c_psi * (ddz + g)) / eta;
    a_ready (3, 2) = term / eta;
    a_ready (3, 3) = 1;

    w_R_b_transpose = w_R_b';
    A_s = w_R_b_transpose * a_ready;

    vector_multiply_to_RT = [-d_psi * s_psi; d_psi * c_psi; 0];
    vector_r_p = [-r; 0; p];
    B_s = (w_R_b_transpose * vector_multiply_to_RT) * d_phi + (vector_r_p * d_theta);

    ph1 = A_s (2, 2) * (d_p - B_s (1));
    ph2 = A_s (1, 2) * (B_s (2) - d_q);
    ph3 = (A_s (1, 2) * A_s (2, 3)) - (A_s (1, 3) * A_s (2, 2));
    ph4 = dd_psi * ph3;

    th1 = A_s (2, 1) * (d_p - B_s (1));
    th2 = A_s (1, 1) * (B_s (2) - d_q);
    th3 = (A_s (1, 1) * A_s (2, 3)) - (A_s (1, 3) * A_s (2, 1));
    th4 = dd_psi * th3;

    den = (A_s (2, 2) * A_s (1, 1)) - (A_s (1, 2) * A_s (2, 1));
    num_ddphi = ph1 + ph2 + ph4;
    num_ddtheta = th4 - th1 - th2;
    dd_phi = num_ddphi / den;
    dd_theta = num_ddtheta / den;

    d_r = B_s (3) + (A_s (3, 1) * dd_phi) + (A_s (3, 2) * dd_theta) + (A_s (3, 3) * dd_psi);

    body_rate = [-p; -q; r];
    body_acc = [-d_p; -d_q; d_r];
    euler = [-phi; -theta; psi];
    euler_rate = [-d_phi; -d_theta; d_psi];
    euler_acc = [-dd_phi; -dd_theta; dd_psi];
    
end

== matlab function INDI_POS_SMC_Att/pos/MATLAB Function2 ==
  data: phi input; theta input; e_p input; tau_Thrust output; e_v input; e_a input; a_ref input; psi_ref input; phi_des output; theta_des output; a_meas input; Thrust_current input; pos_gain parameter size=[3 3]; vel_gain parameter size=[3 3]; acc_gain parameter size=[3 3]; m parameter; Tmax parameter
function [tau_Thrust, phi_des, theta_des] = thrust_and_desired_angles (phi, theta, e_p, e_v, e_a, a_ref, psi_ref, a_meas, Thrust_current, pos_gain, vel_gain, acc_gain, m, Tmax)

a_c = -(pos_gain * e_p) - (vel_gain * e_v) - (acc_gain * e_a) + a_ref;

c_phi = cos (phi);
c_th = cos (theta);


f_c = Thrust_current + (m * (a_c - a_meas));

z_B_des = f_c / norm (f_c);

u_thrust = norm (f_c);

term1 = u_thrust / (4 * c_th * c_phi * Tmax);

tau_Thrust = term1 + 1;
    
u1 = z_B_des(1) * sin(psi_ref) - z_B_des(2) * cos(psi_ref);
u2 = z_B_des(1) * cos(psi_ref) + z_B_des(2) * sin(psi_ref);

phi_des   = atan2(u1, z_B_des(3));
theta_des = atan2(u2, z_B_des(3));

end

== matlab function INDI_POS_SMC_Att/Reference Values/MATLAB Function3 ==
  data: t input; pos output; vel output; acc output; jerk output; snap output
function [pos, vel, acc, jerk, snap] = ref_traj(t)
%#codegen

    pos  = ref_pos(t);
    vel  = ref_vel(t);
    acc  = ref_acc(t);
    jerk = ref_jerk(t);
    snap = ref_snap(t);
end

== matlab function INDI_POS_SMC_Att/Mixer ==
  data: tau_T input; u output; tau_P input; tau_R input; tau_Y input
function u = fcn(tau_T, tau_P, tau_R, tau_Y)

A = [1,  1,  1,  1;
         -1, 1, 1,  -1;
         1,  -1, 1, -1;
         1, 1,  -1, -1];

    b = [4 * tau_T - 4;
        -4 * tau_R;
        -4 * tau_P;
         4 * tau_Y];

    % v1, v2, v3, v4 계산
    u = A \ b;
end
